simulink model "problem_3"  (R2020b)
settings: Solver=VariableStepAuto  StartTime=0.0  StopTime=120  RelTol=1e-3
values from neighbouring files (symbols this model uses):
  b = 50.0    [cruisecontroldata.sldd]    (also in position.sldd = 3.5077E-6)
  m = 1000.0    [cruisecontroldata.sldd]
settings Model: DataDictionary=cruisecontroldata.sldd  OrderedModelArguments=off  Creator=Hp  LastModifiedBy=Hp

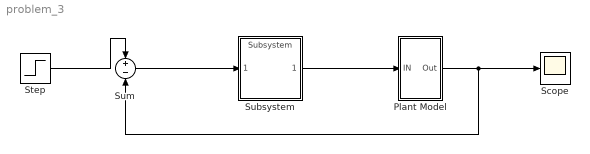
== system problem_3 ==
  Plant Model : Subsystem
  Scope : Scope
  Step : Step  Time=0  After=10  SampleTime=0
  Subsystem : ModelReference  ModelNameDialog=Subsystem  SimulationMode=Normal  ModelReferenceVersion=1.1
  Sum : Sum  Inputs=+-
  wires:
  Plant Model/1(Out) -> Scope/1, Sum/2
  Step/1 -> Sum/1
  Sum/1 -> Subsystem/1
  Subsystem/1 -> Plant Model/1(IN)

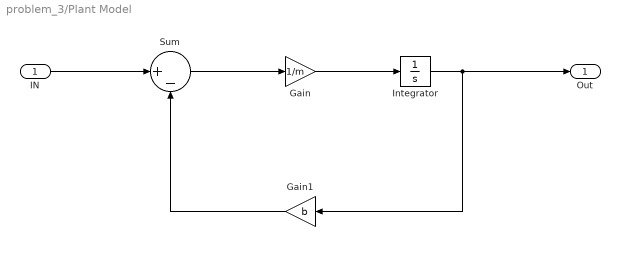
== system problem_3/Plant Model ==
  IN : Inport
  Gain : Gain  Gain=1/m
  Gain1 : Gain  Gain=b
  Integrator : Integrator
  Sum : Sum  Inputs=|+-
  Out : Outport
  wires:
  Gain1/1 -> Sum/2
  Integrator/1 -> Out/1, Gain1/1
  Sum/1 -> Gain/1
  Gain/1 -> Integrator/1
  IN/1 -> Sum/1
